simulink model "Mooventure2016_Rev5"  (Simulink 7.7)
settings: Solver=FixedStepDiscrete  StartTime=0.0  StopTime=10  RelTol=1e-3
PreLoadFcn:
  | try, eval([bdroot '_setup']); catch, eval('model_setup', ''); end
InitFcn:
  | try, eval([bdroot '_setup']); catch, eval('model_setup', ''); end
undefined symbols (not defined in the file): ECM, H1, motohawk_build_version, motohawk_trunc_name, motohawk_vardec_config_group, motohawk_vardec_path, xD
libraries: MotoHawk_lib x976, motohawk_control_primitives_lib x41, simulink x27, motohawk_annotations_lib x3
(part 8 of 16)

== system Mooventure2016_Rev5/Foreground/Control/Battery/Safe Shutdown Sequence ==
  note: This is VERY important to prevent damage to HV system
  note: If battery is present and not shutdown turn on
  note: If shutdown turn off battery load
      | Note: Most of this is managed on output
      | signals of Run/Stop subsystem
  note: 2 Second Delay on battery connect
  Battery Present : Inport  OutDataTypeStr=boolean
  Shutdown Command : Inport  Port=2  OutDataTypeStr=boolean
  Batt Ready : Inport  Port=3  OutDataTypeStr=boolean
  Logical Operator : Logic  Operator=OR  AllPortsSameDT=off  OutDataTypeStr=boolean
  Logical Operator{1,3,5..7} (5 alike) : Logic  Operator=NOT  AllPortsSameDT=off  OutDataTypeStr=boolean
  Logical Operator2 : Logic  AllPortsSameDT=off  OutDataTypeStr=boolean
  Logical Operator4 : Logic  Inputs=3  AllPortsSameDT=off  OutDataTypeStr=boolean
  Logical Operator8 : Logic  Operator=OR  AllPortsSameDT=off  OutDataTypeStr=boolean
  Relational Operator : RelationalOperator  OutDataTypeStr=boolean
  Relational Operator1 : RelationalOperator  OutDataTypeStr=boolean
  Relational Operator2 : RelationalOperator  OutDataTypeStr=boolean
  Time Since Enabled (With Input)1 : motohawk_control_primitives_lib/Time Since Enabled (With Input)1  SystemSampleTime=-1  nam='Contactor_Disable_Timer'  samp_time=-1  init=0  upperlim=3600*24
  Time Since Enabled (With Input)2 : motohawk_control_primitives_lib/Time Since Enabled (With Input)1  SystemSampleTime=-1  nam='Voltage_Filt'  samp_time=-1  init=0  upperlim=3600*24
  Time Since Enabled (With Input)3 : motohawk_control_primitives_lib/Time Since Enabled (With Input)1  SystemSampleTime=-1  nam='Solectria_Enable_timer'  samp_time=-1  init=0  upperlim=3600*24
  motohawk_calibration : MotoHawk_lib/Calibration & Probing Blocks/motohawk_calibration  nam='Contactor_Disable_Delay'  val=0.5  storage=Calibration  show_more=on  name_source=Use Parameter  data_type=Inherit from 'Default Value'  read_level=1  write_level=1  ovr_cals=on  view_as=Number  enum_struct={'Disabled', 'Enabled'}  vector_style=Wide Row  use_help_units=off  help=''  units=''  use_header_enum=off  row_header_enum={}  col_header_enum={}  use_min_max=on  min_val=0  max_val=10  use_precision=on  precision='1.2'  gain=1  offset=0  exp=1  use_mototune_group=on  mototune_group=motohawk_vardec_path(gcb)
  motohawk_calibration1 : MotoHawk_lib/Calibration & Probing Blocks/motohawk_calibration  nam='Load_Enable_Delay'  val=2  storage=Calibration  show_more=on  name_source=Use Parameter  data_type=Inherit from 'Default Value'  read_level=1  write_level=1  ovr_cals=on  view_as=Number  enum_struct={'Disabled', 'Enabled'}  vector_style=Wide Row  use_help_units=off  help=''  units=''  use_header_enum=off  row_header_enum={}  col_header_enum={}  use_min_max=on  min_val=0  max_val=10  use_precision=on  precision='1.2'  gain=1  offset=0  exp=1  use_mototune_group=on  mototune_group=motohawk_vardec_path(gcb)
  motohawk_calibration2 : MotoHawk_lib/Calibration & Probing Blocks/motohawk_calibration  nam='Voltage_Filt_Cal'  val=2  storage=Calibration  show_more=on  name_source=Use Parameter  data_type=Inherit from 'Default Value'  read_level=1  write_level=1  ovr_cals=on  view_as=Number  enum_struct={'Disabled', 'Enabled'}  vector_style=Wide Row  use_help_units=off  help=''  units=''  use_header_enum=off  row_header_enum={}  col_header_enum={}  use_min_max=on  min_val=0  max_val=10  use_precision=on  precision='1.2'  gain=1  offset=0  exp=1  use_mototune_group=on  mototune_group=motohawk_vardec_path(gcb)
  motohawk_data_write : MotoHawk_lib/Data Storage Blocks/motohawk_data_write  source=Lookup By Name  structure=Scalar  operation=Write entire data structure at once  sz_vec=-1  sz_row=3  sz_col=2  typ=boolean  nam='MPRD_KeepAlive'  checkNull=off  write_read_only=off  struct_inst_name='Struct1'  struct_name='MyStruct'
  Contactor_Enable : Outport  OutDataTypeStr=boolean
  Load_Enable : Outport  Port=2  OutDataTypeStr=boolean
  wires:
  Shutdown Command/1 -> Time Since Enabled (With Input)1/1, Logical Operator3/1, Logical Operator5/1
  Time Since Enabled (With Input)1/1 -> Relational Operator/1
  Logical Operator2/1 -> Contactor_Enable/1, Logical Operator/1
  Logical Operator3/1 -> Logical Operator4/1
  Time Since Enabled (With Input)3/1 -> Relational Operator1/1
  Relational Operator1/1 -> Logical Operator4/2
  Logical Operator5/1 -> Time Since Enabled (With Input)3/1
  Logical Operator4/1 -> Load_Enable/1
  motohawk_calibration/1 -> Relational Operator/2
  motohawk_calibration1/1 -> Relational Operator1/2
  Relational Operator/1 -> Logical Operator6/1
  Batt Ready/1 -> Logical Operator4/3
  Logical Operator/1 -> motohawk_data_write/1
  [ReadyLight] -> Logical Operator/2
  Battery Present/1 -> Logical Operator7/1, Logical Operator8/2
  Time Since Enabled (With Input)2/1 -> Relational Operator2/1
  motohawk_calibration2/1 -> Relational Operator2/2
  Relational Operator2/1 -> Logical Operator1/1
  Logical Operator7/1 -> Time Since Enabled (With Input)2/1
  Logical Operator6/1 -> Logical Operator2/2
  Logical Operator8/1 -> Logical Operator2/1
  Logical Operator1/1 -> Logical Operator8/1

== system Mooventure2016_Rev5/Foreground/Control/Engine Control/Engine States ==
  Engine On : Inport
  Product : Product  RndMeth=Zero
  Relational Operator2 : RelationalOperator  OutDataTypeStr=boolean
  Time Since Enabled (With Input)1 : motohawk_control_primitives_lib/Time Since Enabled (With Input)1  SystemSampleTime=-1  nam='Engine_On_Timer'  samp_time=-1  init=0  upperlim=16000
  motohawk_calibration2 : MotoHawk_lib/Calibration & Probing Blocks/motohawk_calibration  nam='Engine_On_Time_Threshold'  val=3  storage=Calibration  show_more=off  name_source=Use Parameter  data_type=Inherit from 'Default Value'  read_level=1  write_level=1  ovr_cals=on  view_as=Number  enum_struct={'Disabled', 'Enabled'}  vector_style=Wide Row  use_help_units=off  help=''  units=''  use_header_enum=off  row_header_enum={}  col_header_enum={}  use_min_max=off  min_val=-inf  max_val=inf  use_precision=off  precision=''  gain=1  offset=0  exp=1  use_mototune_group=off  mototune_group=motohawk_vardec_path(gcb)
  Engine On Out : Outport
  wires:
  Engine On/1 -> Time Since Enabled (With Input)1/1, Product/2
  Time Since Enabled (With Input)1/1 -> Relational Operator2/1
  motohawk_calibration2/1 -> Relational Operator2/2
  Relational Operator2/1 -> Product/1
  Product/1 -> Engine On Out/1

== system Mooventure2016_Rev5/Foreground/Control/Engine Control/SOC States ==
  SOC : Inport
  Product : Product  RndMeth=Zero
  Product1 : Product  RndMeth=Zero
  Product2 : Product  RndMeth=Zero
  Relational Operator : RelationalOperator  Operator=<=  OutDataTypeStr=boolean
  Relational Operator{1..3,5} (4 alike) : RelationalOperator  OutDataTypeStr=boolean
  Relational Operator4 : RelationalOperator  Operator=<=  OutDataTypeStr=boolean
  Time Since Enabled (With Input)1 : motohawk_control_primitives_lib/Time Since Enabled (With Input)1  SystemSampleTime=-1  nam='SOC_Low_Timer'  samp_time=-1  init=0  upperlim=16000
  Time Since Enabled (With Input)2 : motohawk_control_primitives_lib/Time Since Enabled (With Input)1  SystemSampleTime=-1  nam='SOC_High_Timer'  samp_time=-1  init=0  upperlim=16000
  Time Since Enabled (With Input)3 : motohawk_control_primitives_lib/Time Since Enabled (With Input)1  SystemSampleTime=-1  nam='SOC_Critical_Timer'  samp_time=-1  init=0  upperlim=16000
  motohawk_calibration : MotoHawk_lib/Calibration & Probing Blocks/motohawk_calibration  nam='SOC_Low'  val=30  storage=Calibration  show_more=off  name_source=Use Parameter  data_type=Inherit from 'Default Value'  read_level=1  write_level=1  ovr_cals=on  view_as=Number  enum_struct={'Disabled', 'Enabled'}  vector_style=Wide Row  use_help_units=off  help=''  units=''  use_header_enum=off  row_header_enum={}  col_header_enum={}  use_min_max=off  min_val=-inf  max_val=inf  use_precision=off  precision=''  gain=1  offset=0  exp=1  use_mototune_group=off  mototune_group=motohawk_vardec_path(gcb)
  motohawk_calibration1 : MotoHawk_lib/Calibration & Probing Blocks/motohawk_calibration  nam='SOC_High'  val=45  storage=Calibration  show_more=off  name_source=Use Parameter  data_type=Inherit from 'Default Value'  read_level=1  write_level=1  ovr_cals=on  view_as=Number  enum_struct={'Disabled', 'Enabled'}  vector_style=Wide Row  use_help_units=off  help=''  units=''  use_header_enum=off  row_header_enum={}  col_header_enum={}  use_min_max=off  min_val=-inf  max_val=inf  use_precision=off  precision=''  gain=1  offset=0  exp=1  use_mototune_group=off  mototune_group=motohawk_vardec_path(gcb)
  motohawk_calibration2 : MotoHawk_lib/Calibration & Probing Blocks/motohawk_calibration  nam='SOC_Time_Threshold'  val=5  storage=Calibration  show_more=off  name_source=Use Parameter  data_type=Inherit from 'Default Value'  read_level=1  write_level=1  ovr_cals=on  view_as=Number  enum_struct={'Disabled', 'Enabled'}  vector_style=Wide Row  use_help_units=off  help=''  units=''  use_header_enum=off  row_header_enum={}  col_header_enum={}  use_min_max=off  min_val=-inf  max_val=inf  use_precision=off  precision=''  gain=1  offset=0  exp=1  use_mototune_group=off  mototune_group=motohawk_vardec_path(gcb)
  motohawk_calibration3 : MotoHawk_lib/Calibration & Probing Blocks/motohawk_calibration  nam='SOC_Critical'  val=20  storage=Calibration  show_more=off  name_source=Use Parameter  data_type=Inherit from 'Default Value'  read_level=1  write_level=1  ovr_cals=on  view_as=Number  enum_struct={'Disabled', 'Enabled'}  vector_style=Wide Row  use_help_units=off  help=''  units=''  use_header_enum=off  row_header_enum={}  col_header_enum={}  use_min_max=off  min_val=-inf  max_val=inf  use_precision=off  precision=''  gain=1  offset=0  exp=1  use_mototune_group=off  mototune_group=motohawk_vardec_path(gcb)
  SOC Low : Outport
  SOC High : Outport  Port=2
  SOC Critical : Outport  Port=3
  wires:
  SOC/1 -> Relational Operator/1, Relational Operator1/1, Relational Operator4/1
  motohawk_calibration/1 -> Relational Operator/2
  motohawk_calibration1/1 -> Relational Operator1/2
  Relational Operator/1 -> Time Since Enabled (With Input)1/1, Product/2
  Relational Operator1/1 -> Time Since Enabled (With Input)2/1, Product1/2
  Time Since Enabled (With Input)1/1 -> Relational Operator2/1
  Time Since Enabled (With Input)2/1 -> Relational Operator3/1
  motohawk_calibration2/1 -> Relational Operator2/2, Relational Operator3/2, Relational Operator5/2
  motohawk_calibration3/1 -> Relational Operator4/2
  Relational Operator4/1 -> Time Since Enabled (With Input)3/1, Product2/2
  Time Since Enabled (With Input)3/1 -> Relational Operator5/1
  Relational Operator2/1 -> Product/1
  Relational Operator3/1 -> Product1/1
  Relational Operator5/1 -> Product2/1
  Product/1 -> SOC Low/1
  Product1/1 -> SOC High/1
  Product2/1 -> SOC Critical/1

== system Mooventure2016_Rev5/Foreground/Control/Engine Control/Vehicle Speed States ==
  Vehicle Speed : Inport
  Product : Product  RndMeth=Zero
  Product1 : Product  RndMeth=Zero
  Relational Operator : RelationalOperator  OutDataTypeStr=boolean
  Relational Operator1 : RelationalOperator  Operator=<=  OutDataTypeStr=boolean
  Relational Operator2 : RelationalOperator  OutDataTypeStr=boolean
  Relational Operator3 : RelationalOperator  OutDataTypeStr=boolean
  Time Since Enabled (With Input)1 : motohawk_control_primitives_lib/Time Since Enabled (With Input)1  SystemSampleTime=-1  nam='Vehicle_Speed_On_Timer'  samp_time=-1  init=0  upperlim=16000
  Time Since Enabled (With Input)2 : motohawk_control_primitives_lib/Time Since Enabled (With Input)1  SystemSampleTime=-1  nam='Vehicle_Speed_Off_Timer'  samp_time=-1  init=0  upperlim=16000
  motohawk_calibration : MotoHawk_lib/Calibration & Probing Blocks/motohawk_calibration  nam='Vehicle_Speed_On'  val=8  storage=Calibration  show_more=off  name_source=Use Parameter  data_type=Inherit from 'Default Value'  read_level=1  write_level=1  ovr_cals=on  view_as=Number  enum_struct={'Disabled', 'Enabled'}  vector_style=Wide Row  use_help_units=off  help=''  units=''  use_header_enum=off  row_header_enum={}  col_header_enum={}  use_min_max=off  min_val=-inf  max_val=inf  use_precision=off  precision=''  gain=1  offset=0  exp=1  use_mototune_group=off  mototune_group=motohawk_vardec_path(gcb)
  motohawk_calibration1 : MotoHawk_lib/Calibration & Probing Blocks/motohawk_calibration  nam='Vehicle_Speed_Off'  val=3  storage=Calibration  show_more=off  name_source=Use Parameter  data_type=Inherit from 'Default Value'  read_level=1  write_level=1  ovr_cals=on  view_as=Number  enum_struct={'Disabled', 'Enabled'}  vector_style=Wide Row  use_help_units=off  help=''  units=''  use_header_enum=off  row_header_enum={}  col_header_enum={}  use_min_max=off  min_val=-inf  max_val=inf  use_precision=off  precision=''  gain=1  offset=0  exp=1  use_mototune_group=off  mototune_group=motohawk_vardec_path(gcb)
  motohawk_calibration2 : MotoHawk_lib/Calibration & Probing Blocks/motohawk_calibration  nam='Vehicle_Speed_Time_Threshold'  val=3  storage=Calibration  show_more=off  name_source=Use Parameter  data_type=Inherit from 'Default Value'  read_level=1  write_level=1  ovr_cals=on  view_as=Number  enum_struct={'Disabled', 'Enabled'}  vector_style=Wide Row  use_help_units=off  help=''  units=''  use_header_enum=off  row_header_enum={}  col_header_enum={}  use_min_max=off  min_val=-inf  max_val=inf  use_precision=off  precision=''  gain=1  offset=0  exp=1  use_mototune_group=off  mototune_group=motohawk_vardec_path(gcb)
  Speed On : Outport
  Speed Off : Outport  Port=2
  wires:
  Vehicle Speed/1 -> Relational Operator/1, Relational Operator1/1
  motohawk_calibration/1 -> Relational Operator/2
  motohawk_calibration1/1 -> Relational Operator1/2
  Relational Operator/1 -> Time Since Enabled (With Input)1/1, Product/2
  Relational Operator1/1 -> Time Since Enabled (With Input)2/1, Product1/2
  Time Since Enabled (With Input)1/1 -> Relational Operator2/1
  Time Since Enabled (With Input)2/1 -> Relational Operator3/1
  motohawk_calibration2/1 -> Relational Operator2/2, Relational Operator3/2
  Relational Operator3/1 -> Product1/1
  Relational Operator2/1 -> Product/1
  Product/1 -> Speed On/1
  Product1/1 -> Speed Off/1

== system Mooventure2016_Rev5/Foreground/Control/Faults/Accesories ==
  In1 : Inport
  Blend Valves : Subsystem
  Charger : Subsystem
  DC-DC Converter : Subsystem
  HV-Contactors : Subsystem
  HV-Heater System : Subsystem
  motohawk_data_read : MotoHawk_lib/Data Storage Blocks/motohawk_data_read  source=Lookup By Name  structure=Scalar  operation=Read scalar from location by index  sz_vec=4  sz_row=2  sz_col=3  typ=boolean  nam='ChargeEnable'  checkNull=on  struct_inst_name='MyData'  struct_nam='MyStruct'
  wires:
  In1/1 -> Charger/1(In1), DC-DC Converter/1(In1), HV-Heater System/1(In1), Blend Valves/1(In1), HV-Contactors/1(In1)
  motohawk_data_read/1 -> Charger/Enable

== system Mooventure2016_Rev5/Foreground/Control/Faults/Battery ==
  In1 : Inport
  2G BMS & Comms : Subsystem
  Precharge : Subsystem
  Temperature : Subsystem
  wires:
  In1/1 -> Temperature/1(In1), Precharge/1(In1), 2G BMS & Comms/1(In1)

== system Mooventure2016_Rev5/Foreground/Control/Faults/Freeze Frame ==
  In1 : Inport
  Data Write : Subsystem  TreatAsAtomicUnit=on
  motohawk_data_def : MotoHawk_lib/Data Storage Blocks/motohawk_data_def  nam='Freeze_Frame'  container_nam=''  data=[0 0 0 0 0 0; 0 0 0 0 0 0 ]  typ=double  struct_nam='MyStruct'  storage=NonVolatile  outputRef=off  use_vardec=on  window=Display  read_level=1  write_level=1  ovr_cals=on  view_as=Number  enum_struct={'Disabled', 'Enabled'}  vector_style=Wide Row  use_help_units=off  help=''  units=''  use_header_enum=on  row_header_enum=''  col_header_enum={'SYS_TIME', 'Voltage', 'Speed', 'Torque_Request', 'Torque_Delivered', 'Coolant_Temp'}  use_min_max=off  min_val=-inf  max_val=inf  use_precision=off  precision=''  gain=1  offset=0  exp=1  use_mototune_group=off  mototune_group=motohawk_vardec_path(gcb)  eval_name=MyData  data_stores=motohawk_sfun_data_def_data_stores  struct_instances=motohawk_sfun_data_def_struct_instances  vardecs=motohawk_sfun_data_def_vardecs
  motohawk_fault_activity_trigger : MotoHawk_lib/Fault Management Blocks/motohawk_fault_activity_trigger  Tag=Trigger  activity=Active  priority_order=0  inherited=off
  wires:
  motohawk_fault_activity_trigger/1 -> Data Write/Trigger
  In1/1 -> Data Write/1(In1)

== system Mooventure2016_Rev5/Foreground/Control/Faults/Power Train ==
  In1 : Inport
  12V Battery : Subsystem
  Brake Pedal : Subsystem
  Cruise Control : Subsystem
  Electric Motor : Subsystem
  Gas Pedal : Subsystem
  Gear Selector : Subsystem
  Ignition Key : Subsystem
  Traction Control : Subsystem
  Vehicle Speed Sensor : Subsystem
  wires:
  In1/1 -> Vehicle Speed Sensor/1(In1), Cruise Control/1(In1), Gear Selector/1(In1), Gas Pedal/1(In1), Traction Control/1(In1), Electric Motor/1(In1), Brake Pedal/1(In1)

== system Mooventure2016_Rev5/Foreground/Control/Hybrid Control Code/CrawlHomeMode ==
  note: This is brake pedal regen mode
  SoCBounds : Inport
  Inputs : Inport  Port=2
  InReverse : Inport  Port=3
  Action Port : ActionPort  ActionType=case
  Brake Pedal Scaling : Stateflow chart  TreatAsAtomicUnit=on
  Bus Selector : BusSelector  OutputSignals=Driver Inputs.Throttle_Position (signal 5),Driver Inputs.Brake_Position (signal 2)
  Bus Selector1 : BusSelector  OutputSignals=IPT.ID 260 IPT Status 2.IPT_MotorSpeed
  Bus Selector2 : BusSelector  OutputSignals=Battery_Inputs.StateOfCharge
  Chart : Stateflow chart  TreatAsAtomicUnit=on
  Constant : Constant
  Data Type Conversion : DataTypeConversion  OutDataTypeStr=double
  Data Type Conversion1 : DataTypeConversion  OutDataTypeStr=double
  Gas Pedal Scaling : Stateflow chart  TreatAsAtomicUnit=on
  Product : Product  RndMeth=Zero
  Product1 : Product  RndMeth=Zero
  Product2 : Product  RndMeth=Zero
  SOC_RampOut : Subsystem
  Sum : Sum
  motohawk_calibration : MotoHawk_lib/Calibration & Probing Blocks/motohawk_calibration  nam='accelStart_Pedal_safetyMode'  val=.03  storage=Calibration  show_more=off  name_source=Use Parameter  data_type=Inherit from 'Default Value'  read_level=1  write_level=1  ovr_cals=on  view_as=Number  enum_struct={'Disabled', 'Enabled'}  vector_style=Wide Row  use_help_units=off  help=''  units=''  use_header_enum=off  row_header_enum={}  col_header_enum={}  use_min_max=off  min_val=-inf  max_val=inf  use_precision=off  precision=''  gain=1  offset=0  exp=1  use_mototune_group=off  mototune_group=motohawk_vardec_path(gcb)
  motohawk_calibration1 : MotoHawk_lib/Calibration & Probing Blocks/motohawk_calibration  nam='brakeStart_Pedal_safetyMode'  val=.01  storage=Calibration  show_more=off  name_source=Use Parameter  data_type=Inherit from 'Default Value'  read_level=1  write_level=1  ovr_cals=on  view_as=Number  enum_struct={'Disabled', 'Enabled'}  vector_style=Wide Row  use_help_units=off  help=''  units=''  use_header_enum=off  row_header_enum={}  col_header_enum={}  use_min_max=off  min_val=-inf  max_val=inf  use_precision=off  precision=''  gain=1  offset=0  exp=1  use_mototune_group=off  mototune_group=motohawk_vardec_path(gcb)
  motohawk_calibration2 : MotoHawk_lib/Calibration & Probing Blocks/motohawk_calibration  nam='brakeEnd_Pedal_safetyMode'  val=.003  storage=Calibration  show_more=off  name_source=Use Parameter  data_type=Inherit from 'Default Value'  read_level=1  write_level=1  ovr_cals=on  view_as=Number  enum_struct={'Disabled', 'Enabled'}  vector_style=Wide Row  use_help_units=off  help=''  units=''  use_header_enum=off  row_header_enum={}  col_header_enum={}  use_min_max=off  min_val=-inf  max_val=inf  use_precision=off  precision=''  gain=1  offset=0  exp=1  use_mototune_group=off  mototune_group=motohawk_vardec_path(gcb)
  motohawk_calibration3 : MotoHawk_lib/Calibration & Probing Blocks/motohawk_calibration  nam='regenStart_Speed_safetyMode'  val=2  storage=Calibration  show_more=off  name_source=Use Parameter  data_type=Inherit from 'Default Value'  read_level=1  write_level=1  ovr_cals=on  view_as=Number  enum_struct={'Disabled', 'Enabled'}  vector_style=Wide Row  use_help_units=off  help=''  units=''  use_header_enum=off  row_header_enum={}  col_header_enum={}  use_min_max=off  min_val=-inf  max_val=inf  use_precision=off  precision=''  gain=1  offset=0  exp=1  use_mototune_group=off  mototune_group=motohawk_vardec_path(gcb)
  motohawk_calibration4 : MotoHawk_lib/Calibration & Probing Blocks/motohawk_calibration  nam='accelEnd_Pedal_safetyMode'  val=.003  storage=Calibration  show_more=off  name_source=Use Parameter  data_type=Inherit from 'Default Value'  read_level=1  write_level=1  ovr_cals=on  view_as=Number  enum_struct={'Disabled', 'Enabled'}  vector_style=Wide Row  use_help_units=off  help=''  units=''  use_header_enum=off  row_header_enum={}  col_header_enum={}  use_min_max=off  min_val=-inf  max_val=inf  use_precision=off  precision=''  gain=1  offset=0  exp=1  use_mototune_group=off  mototune_group=motohawk_vardec_path(gcb)
  motohawk_calibration5 : MotoHawk_lib/Calibration & Probing Blocks/motohawk_calibration  nam='regenEnd_Speed_safetyMode'  val=0.75  storage=Calibration  show_more=off  name_source=Use Parameter  data_type=Inherit from 'Default Value'  read_level=1  write_level=1  ovr_cals=on  view_as=Number  enum_struct={'Disabled', 'Enabled'}  vector_style=Wide Row  use_help_units=off  help=''  units=''  use_header_enum=off  row_header_enum={}  col_header_enum={}  use_min_max=off  min_val=-inf  max_val=inf  use_precision=off  precision=''  gain=1  offset=0  exp=1  use_mototune_group=off  mototune_group=motohawk_vardec_path(gcb)
  motohawk_calibration6 : MotoHawk_lib/Calibration & Probing Blocks/motohawk_calibration  nam='dragTorque_safetyMode'  val=.028  storage=Calibration  show_more=off  name_source=Use Parameter  data_type=Inherit from 'Default Value'  read_level=1  write_level=1  ovr_cals=on  view_as=Number  enum_struct={'Disabled', 'Enabled'}  vector_style=Wide Row  use_help_units=off  help=''  units=''  use_header_enum=off  row_header_enum={}  col_header_enum={}  use_min_max=off  min_val=-inf  max_val=inf  use_precision=off  precision=''  gain=1  offset=0  exp=1  use_mototune_group=off  mototune_group=motohawk_vardec_path(gcb)
  motohawk_calibration7 : MotoHawk_lib/Calibration & Probing Blocks/motohawk_calibration  nam='RPM_to_Wheel_Speed_Multiplier_safetyMode'  val=0.01001896  storage=Calibration  show_more=off  name_source=Use Parameter  data_type=Inherit from 'Default Value'  read_level=1  write_level=1  ovr_cals=on  view_as=Number  enum_struct={'Disabled', 'Enabled'}  vector_style=Wide Row  use_help_units=off  help=''  units=''  use_header_enum=off  row_header_enum={}  col_header_enum={}  use_min_max=off  min_val=-inf  max_val=inf  use_precision=off  precision=''  gain=1  offset=0  exp=1  use_mototune_group=off  mototune_group=motohawk_vardec_path(gcb)
  motohawk_calibration8 : MotoHawk_lib/Calibration & Probing Blocks/motohawk_calibration  nam='driveMaxTorque_safetyMode'  val=1600  storage=Calibration  show_more=off  name_source=Use Parameter  data_type=Inherit from 'Default Value'  read_level=1  write_level=1  ovr_cals=on  view_as=Number  enum_struct={'Disabled', 'Enabled'}  vector_style=Wide Row  use_help_units=off  help=''  units=''  use_header_enum=off  row_header_enum={}  col_header_enum={}  use_min_max=off  min_val=-inf  max_val=inf  use_precision=off  precision=''  gain=1  offset=0  exp=1  use_mototune_group=off  mototune_group=motohawk_vardec_path(gcb)
  motohawk_calibration9 : MotoHawk_lib/Calibration & Probing Blocks/motohawk_calibration  nam='regenMaxTorque_safetyMode'  val=-300  storage=Calibration  show_more=off  name_source=Use Parameter  data_type=Inherit from 'Default Value'  read_level=1  write_level=1  ovr_cals=on  view_as=Number  enum_struct={'Disabled', 'Enabled'}  vector_style=Wide Row  use_help_units=off  help=''  units=''  use_header_enum=off  row_header_enum={}  col_header_enum={}  use_min_max=off  min_val=-inf  max_val=inf  use_precision=off  precision=''  gain=1  offset=0  exp=1  use_mototune_group=off  mototune_group=motohawk_vardec_path(gcb)
  motohawk_interpolation_1d : MotoHawk_lib/Lookup Tables/motohawk_interpolation_1d  nam='safetyMode_Accel_Map'  table_data=[0:0.05:1]  show_more=on  data_type=double  storage=NonAdaptive  read_level=1  write_level=1  ovr_cals=on  use_help=off  help=''  units=''  use_min_max=off  min_val=0  max_val=1  use_precision=off  precision='1.2'  gain=1  offset=0  exp=1  use_links=on  prelookup_block='safetyMode_Accel'  output_name=''  use_mototune_group=off  mototune_group=motohawk_vardec_path(gcb)
  motohawk_interpolation_1d1 : MotoHawk_lib/Lookup Tables/motohawk_interpolation_1d  nam='safetyMode_Brake_Map'  table_data=[0:0.1:1,1,1,1,1,1,1,1,1,1,1]  show_more=on  data_type=double  storage=NonAdaptive  read_level=1  write_level=1  ovr_cals=on  use_help=off  help=''  units=''  use_min_max=off  min_val=0  max_val=1  use_precision=off  precision='1.2'  gain=1  offset=0  exp=1  use_links=on  prelookup_block='safetyMode_Brake'  output_name=''  use_mototune_group=off  mototune_group=motohawk_vardec_path(gcb)
  motohawk_prelookup : MotoHawk_lib/Lookup Tables/motohawk_prelookup  nam='safetyMode_Accel'  breakpoint_data=[0:0.05:1]  show_more=on  data_type=double  storage=Constant  read_level=1  write_level=1  ovr_cals=on  use_help=off  help=''  units=''  use_min_max=off  min_val=-inf  max_val=inf  use_precision=off  precision=''  gain=1  offset=0  exp=1  use_links=off  input_name=''  use_mototune_group=off  mototune_group=motohawk_vardec_path(gcb)
  motohawk_prelookup1 : MotoHawk_lib/Lookup Tables/motohawk_prelookup  nam='safetyMode_Brake'  breakpoint_data=[0:0.05:1]  show_more=on  data_type=double  storage=Constant  read_level=1  write_level=1  ovr_cals=on  use_help=off  help=''  units=''  use_min_max=off  min_val=-inf  max_val=inf  use_precision=off  precision=''  gain=1  offset=0  exp=1  use_links=off  input_name=''  use_mototune_group=off  mototune_group=motohawk_vardec_path(gcb)
  motohawk_probe : MotoHawk_lib/Calibration & Probing Blocks/motohawk_probe  nam='Gas_Pedal_Prb_safetyMode'  show_more=off  name_source=Use Parameter  read_level=1  view_as=Number  enum_struct={'Disabled', 'Enabled'}  vector_style=Wide Row  use_help_units=off  help=''  units=''  use_header_enum=off  row_header_enum={}  col_header_enum={}  use_precision=off  precision=''  gain=1  offset=0  exp=1  use_mototune_group=off  mototune_group=motohawk_vardec_path(gcb)
  motohawk_probe1 : MotoHawk_lib/Calibration & Probing Blocks/motohawk_probe  nam='driveTorque_Prb_safetyMode'  show_more=off  name_source=Use Parameter  read_level=1  view_as=Number  enum_struct={'Disabled', 'Enabled'}  vector_style=Wide Row  use_help_units=off  help=''  units=''  use_header_enum=off  row_header_enum={}  col_header_enum={}  use_precision=off  precision=''  gain=1  offset=0  exp=1  use_mototune_group=off  mototune_group=motohawk_vardec_path(gcb)
  motohawk_probe2 : MotoHawk_lib/Calibration & Probing Blocks/motohawk_probe  nam='Brake_Pedal_Prb_safetyMode'  show_more=off  name_source=Use Parameter  read_level=1  view_as=Number  enum_struct={'Disabled', 'Enabled'}  vector_style=Wide Row  use_help_units=off  help=''  units=''  use_header_enum=off  row_header_enum={}  col_header_enum={}  use_precision=off  precision=''  gain=1  offset=0  exp=1  use_mototune_group=off  mototune_group=motohawk_vardec_path(gcb)
  motohawk_probe3 : MotoHawk_lib/Calibration & Probing Blocks/motohawk_probe  nam='regenTorque_Prb_safetyMode'  show_more=off  name_source=Use Parameter  read_level=1  view_as=Number  enum_struct={'Disabled', 'Enabled'}  vector_style=Wide Row  use_help_units=off  help=''  units=''  use_header_enum=off  row_header_enum={}  col_header_enum={}  use_precision=off  precision=''  gain=1  offset=0  exp=1  use_mototune_group=off  mototune_group=motohawk_vardec_path(gcb)
  Motor Torque : Outport  InitialOutput=0
  Motor Enable : Outport  Port=2  InitialOutput=0
  wires:
  SOC_RampOut/1(Torque_Out) -> Motor Torque/1
  SoCBounds/1 -> SOC_RampOut/3(SoCBounds)
  Bus Selector2/1 -> SOC_RampOut/2(SOC)  "<StateOfCharge>"
  Inputs/1 -> Bus Selector/1, Bus Selector1/1, Bus Selector2/1
  Bus Selector/1 -> Data Type Conversion/1  "<Throttle_Position (signal 5)>"
  Constant/1 -> Motor Enable/1
  Data Type Conversion/1 -> Gas Pedal Scaling/1(throttleIn)  "motor_Torque"
  Gas Pedal Scaling/1(throttleOut) -> motohawk_probe/1, motohawk_prelookup/1  "motor_Torque"
  Data Type Conversion1/1 -> Brake Pedal Scaling/1(brakeIn)
  Brake Pedal Scaling/1(brakeOut) -> motohawk_probe2/1, motohawk_prelookup1/1  "Brake_Pedal"
  InReverse/1 -> Brake Pedal Scaling/2(inReverse)
  Bus Selector/2 -> Data Type Conversion1/1  "<Brake_Position (signal 2)>"
  motohawk_prelookup/1 -> motohawk_interpolation_1d/1
  motohawk_prelookup1/1 -> motohawk_interpolation_1d1/1
  Bus Selector1/1 -> Product/2  "<IPT_MotorSpeed>"
  motohawk_calibration7/1 -> Product/1
  motohawk_interpolation_1d/1 -> Chart/1(accel)
  motohawk_interpolation_1d1/1 -> Chart/2(brake)
  Product/1 -> Chart/3(speed)
  motohawk_calibration/1 -> Chart/4(accelStart)
  motohawk_calibration4/1 -> Chart/5(accelEnd)
  motohawk_calibration1/1 -> Chart/6(brakeStart)
  motohawk_calibration2/1 -> Chart/7(brakeEnd)
  motohawk_calibration3/1 -> Chart/8(regenStart)
  motohawk_calibration5/1 -> Chart/9(regenEnd)
  motohawk_calibration6/1 -> Chart/10(dragTorque)
  Chart/1(driveTorque) -> Product1/1, motohawk_probe1/1
  Chart/2(regenTorque) -> Product2/1, motohawk_probe3/1
  Product1/1 -> Sum/1
  Product2/1 -> Sum/2
  Sum/1 -> SOC_RampOut/1(Torque_In)
  motohawk_calibration8/1 -> Product1/2
  motohawk_calibration9/1 -> Product2/2

== system Mooventure2016_Rev5/Foreground/Control/Hybrid Control Code/Cruise Control ==
  Inputs : Inport
  Torque : Inport  Port=2
  Brake Disable : Subsystem  TreatAsAtomicUnit=on
  Bus Creator : BusCreator  Inputs=1
  Bus Selector : BusSelector  OutputSignals=IPT.ID 260 IPT Status 2.IPT_MotorSpeed,Cruise Control.Set-,Cruise Control.Set+,Cruise Control.RSM,Cruise Control.Off,Cruise Control.ON,Driver Inputs.Brake_Position (signal 2)
  Logical Operator : Logic  Operator=OR  AllPortsSameDT=off  OutDataTypeStr=boolean
  Logical Operator1 : Logic  Inputs=4  AllPortsSameDT=off  OutDataTypeStr=boolean
  Logical Operator2 : Logic  Operator=NOT  AllPortsSameDT=off  OutDataTypeStr=boolean
  Logical Operator3 : Logic  AllPortsSameDT=off  OutDataTypeStr=boolean
  Logical Operator4 : Logic  Operator=NOT  AllPortsSameDT=off  OutDataTypeStr=boolean
  Logical Operator5 : Logic  AllPortsSameDT=off  OutDataTypeStr=boolean
  Product : Product  RndMeth=Zero
  Product1 : Product  RndMeth=Zero
  Relational Operator : RelationalOperator  OutDataTypeStr=boolean
  Relational Operator1 : RelationalOperator  Operator=<  OutDataTypeStr=boolean
  Speed Changing : Subsystem
  Speed Control : Subsystem
  Speed Resume : Subsystem
  System Start : Subsystem  TreatAsAtomicUnit=on
  SystemState : Stateflow chart  TreatAsAtomicUnit=on
  motohawk_calibration : MotoHawk_lib/Calibration & Probing Blocks/motohawk_calibration  nam='Cruise_Control_Enable'  val=0  storage=Calibration  show_more=off  name_source=Use Parameter  data_type=Inherit from 'Default Value'  read_level=1  write_level=1  ovr_cals=on  view_as=Number  enum_struct={'Disabled', 'Enabled'}  vector_style=Wide Row  use_help_units=off  help=''  units=''  use_header_enum=off  row_header_enum={}  col_header_enum={}  use_min_max=off  min_val=-inf  max_val=inf  use_precision=off  precision=''  gain=1  offset=0  exp=1  use_mototune_group=off  mototune_group=motohawk_vardec_path(gcb)
  motohawk_calibration1 : MotoHawk_lib/Calibration & Probing Blocks/motohawk_calibration  nam='Cruise_On_Speed'  val=25  storage=Calibration  show_more=off  name_source=Use Parameter  data_type=Inherit from 'Default Value'  read_level=1  write_level=1  ovr_cals=on  view_as=Number  enum_struct={'Disabled', 'Enabled'}  vector_style=Wide Row  use_help_units=off  help=''  units=''  use_header_enum=off  row_header_enum={}  col_header_enum={}  use_min_max=off  min_val=-inf  max_val=inf  use_precision=off  precision=''  gain=1  offset=0  exp=1  use_mototune_group=off  mototune_group=motohawk_vardec_path(gcb)
  motohawk_calibration2 : MotoHawk_lib/Calibration & Probing Blocks/motohawk_calibration  nam='Cruise_Disable_Brake'  val=32800  storage=Calibration  show_more=off  name_source=Use Parameter  data_type=Inherit from 'Default Value'  read_level=1  write_level=1  ovr_cals=on  view_as=Number  enum_struct={'Disabled', 'Enabled'}  vector_style=Wide Row  use_help_units=off  help=''  units=''  use_header_enum=off  row_header_enum={}  col_header_enum={}  use_min_max=off  min_val=-inf  max_val=inf  use_precision=off  precision=''  gain=1  offset=0  exp=1  use_mototune_group=off  mototune_group=motohawk_vardec_path(gcb)
  motohawk_calibration7 : MotoHawk_lib/Calibration & Probing Blocks/motohawk_calibration  nam='MPH_Conversion'  val=0.01001896  storage=Calibration  show_more=off  name_source=Use Parameter  data_type=Inherit from 'Default Value'  read_level=1  write_level=1  ovr_cals=on  view_as=Number  enum_struct={'Disabled', 'Enabled'}  vector_style=Wide Row  use_help_units=off  help=''  units=''  use_header_enum=off  row_header_enum={}  col_header_enum={}  use_min_max=off  min_val=-inf  max_val=inf  use_precision=off  precision=''  gain=1  offset=0  exp=1  use_mototune_group=off  mototune_group=motohawk_vardec_path(gcb)
  motohawk_data_def : MotoHawk_lib/Data Storage Blocks/motohawk_data_def  nam='CruiseSpeed'  container_nam=''  data=0  typ=double  struct_nam='MyStruct'  storage=Volatile  outputRef=off  use_vardec=off  window=Display  read_level=1  write_level=1  ovr_cals=on  view_as=Number  enum_struct={'Disabled', 'Enabled'}  vector_style=Wide Row  use_help_units=off  help=''  units=''  use_header_enum=off  row_header_enum=''  col_header_enum=''  use_min_max=off  min_val=-inf  max_val=inf  use_precision=off  precision=''  gain=1  offset=0  exp=1  use_mototune_group=off  mototune_group=motohawk_vardec_path(gcb)  eval_name=MyData  data_stores=motohawk_sfun_data_def_data_stores  struct_instances=motohawk_sfun_data_def_struct_instances  vardecs=motohawk_sfun_data_def_vardecs
  motohawk_data_def1 : MotoHawk_lib/Data Storage Blocks/motohawk_data_def  nam='CruiseOn'  container_nam=''  data=0  typ=boolean  struct_nam='MyStruct'  storage=Volatile  outputRef=off  use_vardec=off  window=Display  read_level=1  write_level=1  ovr_cals=on  view_as=Number  enum_struct={'Disabled', 'Enabled'}  vector_style=Wide Row  use_help_units=off  help=''  units=''  use_header_enum=off  row_header_enum=''  col_header_enum=''  use_min_max=off  min_val=-inf  max_val=inf  use_precision=off  precision=''  gain=1  offset=0  exp=1  use_mototune_group=off  mototune_group=motohawk_vardec_path(gcb)  eval_name=MyData  data_stores=motohawk_sfun_data_def_data_stores  struct_instances=motohawk_sfun_data_def_struct_instances  vardecs=motohawk_sfun_data_def_vardecs
  motohawk_data_read : MotoHawk_lib/Data Storage Blocks/motohawk_data_read  source=Lookup By Name  structure=Scalar  operation=Read scalar from location by index  sz_vec=4  sz_row=2  sz_col=3  typ=boolean  nam='CruiseOn'  checkNull=on  struct_inst_name='MyData'  struct_nam='MyStruct'
  motohawk_data_read1 : MotoHawk_lib/Data Storage Blocks/motohawk_data_read  source=Lookup By Name  structure=Scalar  operation=Read scalar from location by index  sz_vec=4  sz_row=2  sz_col=3  typ=boolean  nam='CruiseOn'  checkNull=on  struct_inst_name='MyData'  struct_nam='MyStruct'
  motohawk_data_read2 : MotoHawk_lib/Data Storage Blocks/motohawk_data_read  source=Lookup By Name  structure=Scalar  operation=Read scalar from location by index  sz_vec=4  sz_row=2  sz_col=3  typ=double  nam='CruiseSpeed'  checkNull=on  struct_inst_name='MyData'  struct_nam='MyStruct'
  motohawk_fault_action3 : MotoHawk_lib/Fault Management Blocks/motohawk_fault_action  nam='Cruise'  output_status=on  eval_nam=Cruise
  Outputs : Outport
  TorqueOut : Outport  Port=2
  wires:
  Inputs/1 -> Bus Selector/1
  Bus Selector/5 -> SystemState/1(CruiseOff)  "<Off>"
  Bus Selector/6 -> SystemState/2(CruiseOn)  "<ON>"
  Torque/1 -> Speed Control/1(Torque)
  Speed Control/1(TorqueOut) -> TorqueOut/1
  SystemState/1(System) -> Logical Operator1/3, Bus Creator/1, Logical Operator3/2  "CruiseLight"
  Bus Creator/1 -> Outputs/1
  Bus Selector/1 -> Product/1  "<IPT_MotorSpeed>"
  motohawk_calibration7/1 -> Product/2
  Bus Selector/2 -> Logical Operator/1, Speed Changing/1(Set-)  "<Set->"
  Bus Selector/3 -> Logical Operator/2, Speed Changing/2(Set+)  "<Set+>"
  Product/1 -> Relational Operator/1, Speed Control/2(CurrentSpeed), Product1/1
  motohawk_calibration1/1 -> Relational Operator/2
  Logical Operator/1 -> Logical Operator1/2
  Relational Operator/1 -> Logical Operator1/1
  Logical Operator1/1 -> Product1/2, System Start/Enable
  Product1/1 -> System Start/1(In1)
  motohawk_data_read/1 -> Logical Operator2/1
  Logical Operator2/1 -> Logical Operator1/4
  Logical Operator3/1 -> Speed Control/4(SystemEnable)
  motohawk_data_read1/1 -> Logical Operator3/1
  motohawk_data_read2/1 -> Speed Control/3(DesiredSpeed)
  Bus Selector/4 -> Speed Resume/1(In1)  "<RSM>"
  Bus Selector/7 -> Relational Operator1/1  "<Brake_Position (signal 2)>"
  motohawk_calibration2/1 -> Relational Operator1/2
  Relational Operator1/1 -> Brake Disable/Enable
  motohawk_fault_action3/1 -> Logical Operator4/1
  motohawk_calibration/1 -> Logical Operator5/1
  Logical Operator4/1 -> Logical Operator5/2
  Logical Operator5/1 -> SystemState/3(CruiseEnable)
